simulink model "TST_VehV_DD"  (R2016b)
settings: Solver=FixedStepDiscrete  StartTime=0.0  StopTime=simTime  FixedStep=sampleTime  RelTol=1e-3
values from neighbouring files (symbols this model uses):
  testCase = 1    [initTST_VehV_DD_001.m]    (also in initTST_VehV_DD_002.m = 2)
libraries: simulink x3
settings Model: Creator=胡炎林  LastModifiedBy=胡炎林
settings DebuggingCC: SignalRangeChecking=error

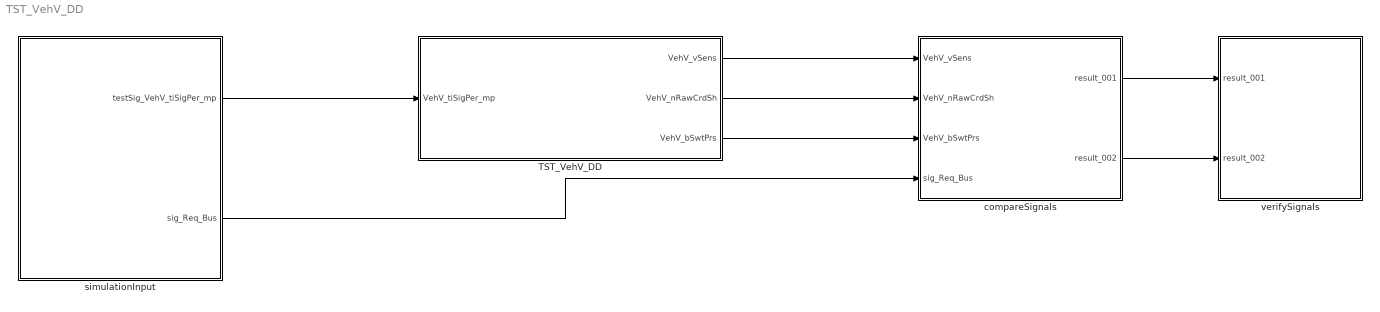
== system TST_VehV_DD ==
  TST_VehV_DD : Subsystem
  compareSignals : Subsystem
  simulationInput : Subsystem
  verifySignals : Subsystem
  wires:
  simulationInput/1(testSig_VehV_tiSigPer_mp) -> TST_VehV_DD/1(VehV_tiSigPer_mp)
  TST_VehV_DD/1(VehV_vSens) -> compareSignals/1(VehV_vSens)
  TST_VehV_DD/2(VehV_nRawCrdSh) -> compareSignals/2(VehV_nRawCrdSh)
  TST_VehV_DD/3(VehV_bSwtPrs) -> compareSignals/3(VehV_bSwtPrs)
  simulationInput/2(sig_Req_Bus) -> compareSignals/4(sig_Req_Bus)
  compareSignals/1(result_001) -> verifySignals/1(result_001)
  compareSignals/2(result_002) -> verifySignals/2(result_002)

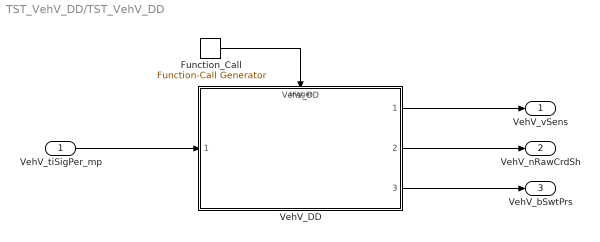
== system TST_VehV_DD/TST_VehV_DD ==
  VehV_tiSigPer_mp : Inport
  Function_Call : simulink/Ports & Subsystems/Function-Call Generator  sample_time=sampleTime  numberOfIterations=1
  VehV_DD : ModelReference  ModelNameDialog=VehV_DD  ModelReferenceVersion=1.6  TriggerPortName=function  TriggerPortTriggerType=function-call  TriggerPortStatesWhenEnabling=held
  VehV_vSens : Outport
  VehV_nRawCrdSh : Outport  Port=2
  VehV_bSwtPrs : Outport  Port=3
  wires:
  Function_Call/1 -> VehV_DD/Trigger
  VehV_tiSigPer_mp/1 -> VehV_DD/1
  VehV_DD/1 -> VehV_vSens/1
  VehV_DD/2 -> VehV_nRawCrdSh/1
  VehV_DD/3 -> VehV_bSwtPrs/1

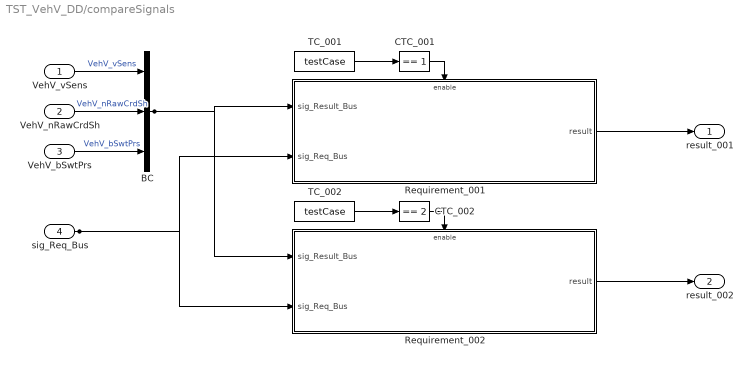
== system TST_VehV_DD/compareSignals ==
  VehV_vSens : Inport
  VehV_nRawCrdSh : Inport  Port=2
  VehV_bSwtPrs : Inport  Port=3
  sig_Req_Bus : Inport  Port=4
  BC : BusCreator  Inputs=3
  CTC_001 : simulink/Logic and Bit Operations/Compare To Constant  relop===  const=1  OutDataTypeStr=boolean
  CTC_002 : simulink/Logic and Bit Operations/Compare To Constant  relop===  const=2  OutDataTypeStr=boolean
  Requirement_001 : Subsystem
  Requirement_002 : Subsystem
  TC_001 : Constant  Value=testCase
  TC_002 : Constant  Value=testCase
  result_001 : Outport
  result_002 : Outport  Port=2
  wires:
  VehV_vSens/1 -> BC/1  "VehV_vSens"
  VehV_nRawCrdSh/1 -> BC/2  "VehV_nRawCrdSh"
  VehV_bSwtPrs/1 -> BC/3  "VehV_bSwtPrs"
  TC_001/1 -> CTC_001/1
  CTC_001/1 -> Requirement_001/Enable
  sig_Req_Bus/1 -> Requirement_001/2(sig_Req_Bus), Requirement_002/2(sig_Req_Bus)
  BC/1 -> Requirement_001/1(sig_Result_Bus), Requirement_002/1(sig_Result_Bus)
  Requirement_001/1(result) -> result_001/1
  TC_002/1 -> CTC_002/1
  CTC_002/1 -> Requirement_002/Enable
  Requirement_002/1(result) -> result_002/1

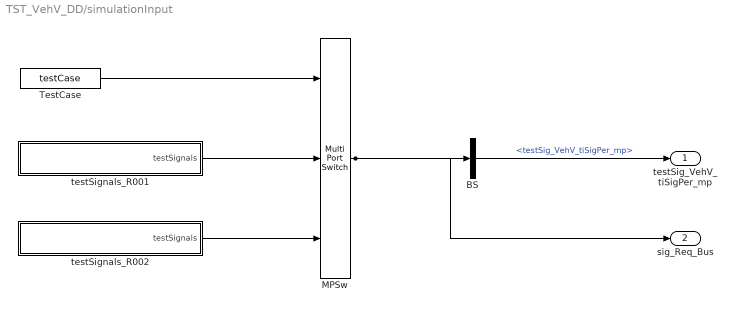
== system TST_VehV_DD/simulationInput ==
  BS : BusSelector  OutputSignals=testSig_VehV_tiSigPer_mp
  MPSw : MultiPortSwitch  Inputs=2  SaturateOnIntegerOverflow=on  InputSameDT=on
  TestCase : Constant  Value=testCase
  testSignals_R001 : Subsystem
  testSignals_R002 : Subsystem
  testSig_VehV_tiSigPer_mp : Outport
  sig_Req_Bus : Outport  Port=2
  wires:
  BS/1 -> testSig_VehV_tiSigPer_mp/1  "<testSig_VehV_tiSigPer_mp>"
  MPSw/1 -> BS/1, sig_Req_Bus/1
  TestCase/1 -> MPSw/1
  testSignals_R001/1(testSignals) -> MPSw/2
  testSignals_R002/1(testSignals) -> MPSw/3

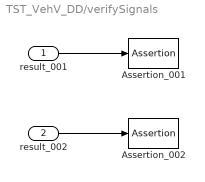
== system TST_VehV_DD/verifySignals ==
  result_001 : Inport
  result_002 : Inport  Port=2
  Assertion_001 : Assertion  Enabled=off
  Assertion_002 : Assertion  Enabled=off
  wires:
  result_001/1 -> Assertion_001/1
  result_002/1 -> Assertion_002/1

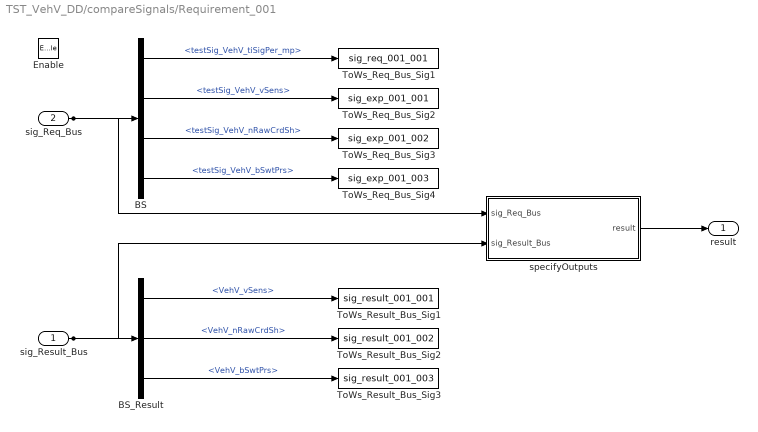
== system TST_VehV_DD/compareSignals/Requirement_001 ==
  sig_Result_Bus : Inport
  sig_Req_Bus : Inport  Port=2
  Enable : EnablePort
  BS : BusSelector  OutputSignals=testSig_VehV_tiSigPer_mp,testSig_VehV_vSens,testSig_VehV_nRawCrdSh,testSig_VehV_bSwtPrs
  BS_Result : BusSelector  OutputSignals=VehV_vSens,VehV_nRawCrdSh,VehV_bSwtPrs
  ToWs_Req_Bus_Sig1 : ToWorkspace  VariableName=sig_req_001_001  SaveFormat=Structure With Time
  ToWs_Req_Bus_Sig2 : ToWorkspace  VariableName=sig_exp_001_001  SaveFormat=Structure With Time
  ToWs_Req_Bus_Sig3 : ToWorkspace  VariableName=sig_exp_001_002  SaveFormat=Structure With Time
  ToWs_Req_Bus_Sig4 : ToWorkspace  VariableName=sig_exp_001_003  SaveFormat=Structure With Time
  ToWs_Result_Bus_Sig1 : ToWorkspace  VariableName=sig_result_001_001  SaveFormat=Structure With Time
  ToWs_Result_Bus_Sig2 : ToWorkspace  VariableName=sig_result_001_002  SaveFormat=Structure With Time
  ToWs_Result_Bus_Sig3 : ToWorkspace  VariableName=sig_result_001_003  SaveFormat=Structure With Time
  specifyOutputs : Subsystem
  result : Outport
  wires:
  sig_Req_Bus/1 -> BS/1, specifyOutputs/1(sig_Req_Bus)
  BS/1 -> ToWs_Req_Bus_Sig1/1  "<testSig_VehV_tiSigPer_mp>"
  BS/2 -> ToWs_Req_Bus_Sig2/1  "<testSig_VehV_vSens>"
  BS/3 -> ToWs_Req_Bus_Sig3/1  "<testSig_VehV_nRawCrdSh>"
  BS/4 -> ToWs_Req_Bus_Sig4/1  "<testSig_VehV_bSwtPrs>"
  sig_Result_Bus/1 -> BS_Result/1, specifyOutputs/2(sig_Result_Bus)
  BS_Result/1 -> ToWs_Result_Bus_Sig1/1  "<VehV_vSens>"
  BS_Result/2 -> ToWs_Result_Bus_Sig2/1  "<VehV_nRawCrdSh>"
  BS_Result/3 -> ToWs_Result_Bus_Sig3/1  "<VehV_bSwtPrs>"
  specifyOutputs/1(result) -> result/1

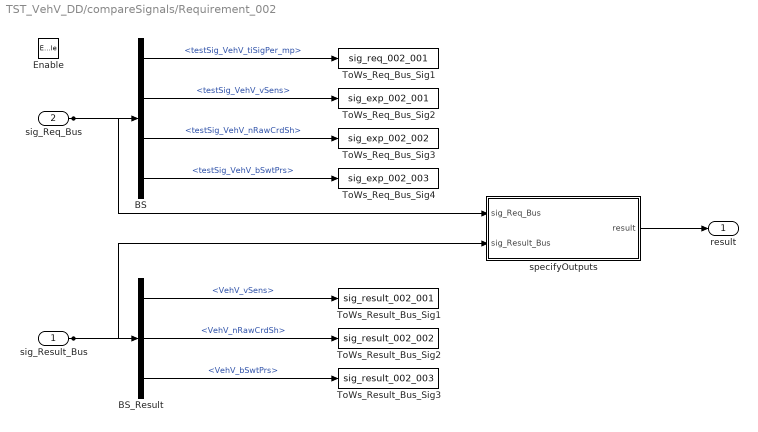
== system TST_VehV_DD/compareSignals/Requirement_002 ==
  sig_Result_Bus : Inport
  sig_Req_Bus : Inport  Port=2
  Enable : EnablePort
  BS : BusSelector  OutputSignals=testSig_VehV_tiSigPer_mp,testSig_VehV_vSens,testSig_VehV_nRawCrdSh,testSig_VehV_bSwtPrs
  BS_Result : BusSelector  OutputSignals=VehV_vSens,VehV_nRawCrdSh,VehV_bSwtPrs
  ToWs_Req_Bus_Sig1 : ToWorkspace  VariableName=sig_req_002_001  SaveFormat=Structure With Time
  ToWs_Req_Bus_Sig2 : ToWorkspace  VariableName=sig_exp_002_001  SaveFormat=Structure With Time
  ToWs_Req_Bus_Sig3 : ToWorkspace  VariableName=sig_exp_002_002  SaveFormat=Structure With Time
  ToWs_Req_Bus_Sig4 : ToWorkspace  VariableName=sig_exp_002_003  SaveFormat=Structure With Time
  ToWs_Result_Bus_Sig1 : ToWorkspace  VariableName=sig_result_002_001  SaveFormat=Structure With Time
  ToWs_Result_Bus_Sig2 : ToWorkspace  VariableName=sig_result_002_002  SaveFormat=Structure With Time
  ToWs_Result_Bus_Sig3 : ToWorkspace  VariableName=sig_result_002_003  SaveFormat=Structure With Time
  specifyOutputs : Subsystem
  result : Outport
  wires:
  sig_Req_Bus/1 -> BS/1, specifyOutputs/1(sig_Req_Bus)
  BS/1 -> ToWs_Req_Bus_Sig1/1  "<testSig_VehV_tiSigPer_mp>"
  BS/2 -> ToWs_Req_Bus_Sig2/1  "<testSig_VehV_vSens>"
  BS/3 -> ToWs_Req_Bus_Sig3/1  "<testSig_VehV_nRawCrdSh>"
  BS/4 -> ToWs_Req_Bus_Sig4/1  "<testSig_VehV_bSwtPrs>"
  sig_Result_Bus/1 -> BS_Result/1, specifyOutputs/2(sig_Result_Bus)
  BS_Result/1 -> ToWs_Result_Bus_Sig1/1  "<VehV_vSens>"
  BS_Result/2 -> ToWs_Result_Bus_Sig2/1  "<VehV_nRawCrdSh>"
  BS_Result/3 -> ToWs_Result_Bus_Sig3/1  "<VehV_bSwtPrs>"
  specifyOutputs/1(result) -> result/1

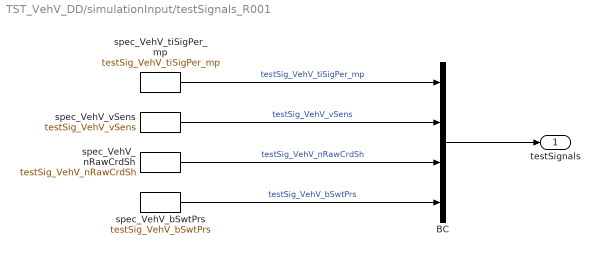
== system TST_VehV_DD/simulationInput/testSignals_R001 ==
  BC : BusCreator  Inputs=4
  spec_VehV_bSwtPrs : FromWorkspace  VariableName=testSig_VehV_bSwtPrs  Interpolate=off  OutputAfterFinalValue=Holding final value
  spec_VehV_nRawCrdSh : FromWorkspace  VariableName=testSig_VehV_nRawCrdSh  Interpolate=off  OutputAfterFinalValue=Holding final value
  spec_VehV_tiSigPer_mp : FromWorkspace  VariableName=testSig_VehV_tiSigPer_mp  Interpolate=off  OutputAfterFinalValue=Holding final value
  spec_VehV_vSens : FromWorkspace  VariableName=testSig_VehV_vSens  Interpolate=off  OutputAfterFinalValue=Holding final value
  testSignals : Outport
  wires:
  BC/1 -> testSignals/1
  spec_VehV_tiSigPer_mp/1 -> BC/1  "testSig_VehV_tiSigPer_mp"
  spec_VehV_vSens/1 -> BC/2  "testSig_VehV_vSens"
  spec_VehV_nRawCrdSh/1 -> BC/3  "testSig_VehV_nRawCrdSh"
  spec_VehV_bSwtPrs/1 -> BC/4  "testSig_VehV_bSwtPrs"

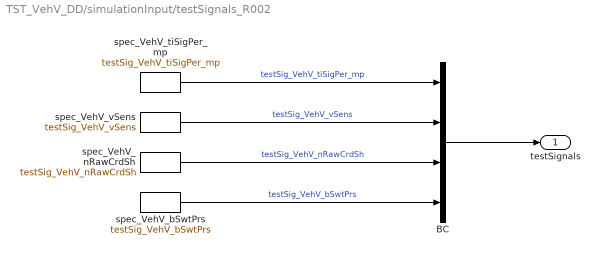
== system TST_VehV_DD/simulationInput/testSignals_R002 ==
  BC : BusCreator  Inputs=4
  spec_VehV_bSwtPrs : FromWorkspace  VariableName=testSig_VehV_bSwtPrs  Interpolate=off  OutputAfterFinalValue=Holding final value
  spec_VehV_nRawCrdSh : FromWorkspace  VariableName=testSig_VehV_nRawCrdSh  Interpolate=off  OutputAfterFinalValue=Holding final value
  spec_VehV_tiSigPer_mp : FromWorkspace  VariableName=testSig_VehV_tiSigPer_mp  Interpolate=off  OutputAfterFinalValue=Holding final value
  spec_VehV_vSens : FromWorkspace  VariableName=testSig_VehV_vSens  Interpolate=off  OutputAfterFinalValue=Holding final value
  testSignals : Outport
  wires:
  BC/1 -> testSignals/1
  spec_VehV_tiSigPer_mp/1 -> BC/1  "testSig_VehV_tiSigPer_mp"
  spec_VehV_vSens/1 -> BC/2  "testSig_VehV_vSens"
  spec_VehV_nRawCrdSh/1 -> BC/3  "testSig_VehV_nRawCrdSh"
  spec_VehV_bSwtPrs/1 -> BC/4  "testSig_VehV_bSwtPrs"

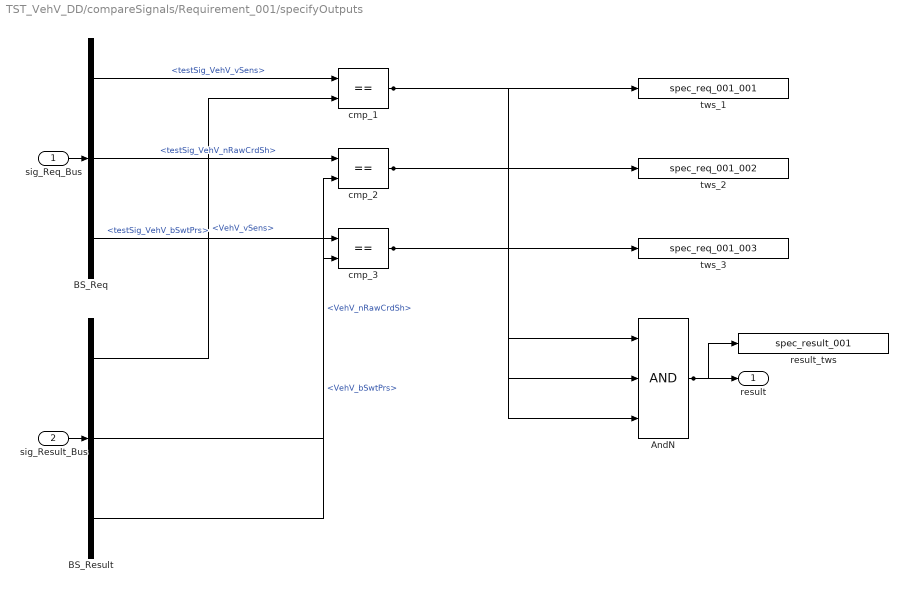
== system TST_VehV_DD/compareSignals/Requirement_001/specifyOutputs ==
  sig_Req_Bus : Inport
  sig_Result_Bus : Inport  Port=2
  AndN : Logic  Inputs=3
  BS_Req : BusSelector  OutputSignals=testSig_VehV_vSens,testSig_VehV_nRawCrdSh,testSig_VehV_bSwtPrs
  BS_Result : BusSelector  OutputSignals=VehV_vSens,VehV_nRawCrdSh,VehV_bSwtPrs
  cmp_1 : RelationalOperator  Operator===  RndMeth=Nearest  InputSameDT=on
  cmp_2 : RelationalOperator  Operator===  RndMeth=Nearest  InputSameDT=on
  cmp_3 : RelationalOperator  Operator===  RndMeth=Nearest  InputSameDT=on
  result_tws : ToWorkspace  VariableName=spec_result_001
  tws_1 : ToWorkspace  VariableName=spec_req_001_001
  tws_2 : ToWorkspace  VariableName=spec_req_001_002
  tws_3 : ToWorkspace  VariableName=spec_req_001_003
  result : Outport
  wires:
  sig_Req_Bus/1 -> BS_Req/1
  sig_Result_Bus/1 -> BS_Result/1
  AndN/1 -> result/1, result_tws/1
  BS_Req/1 -> cmp_1/1  "<testSig_VehV_vSens>"
  BS_Result/1 -> cmp_1/2  "<VehV_vSens>"
  cmp_1/1 -> tws_1/1, AndN/1
  BS_Req/2 -> cmp_2/1  "<testSig_VehV_nRawCrdSh>"
  BS_Result/2 -> cmp_2/2  "<VehV_nRawCrdSh>"
  cmp_2/1 -> tws_2/1, AndN/2
  BS_Req/3 -> cmp_3/1  "<testSig_VehV_bSwtPrs>"
  BS_Result/3 -> cmp_3/2  "<VehV_bSwtPrs>"
  cmp_3/1 -> tws_3/1, AndN/3

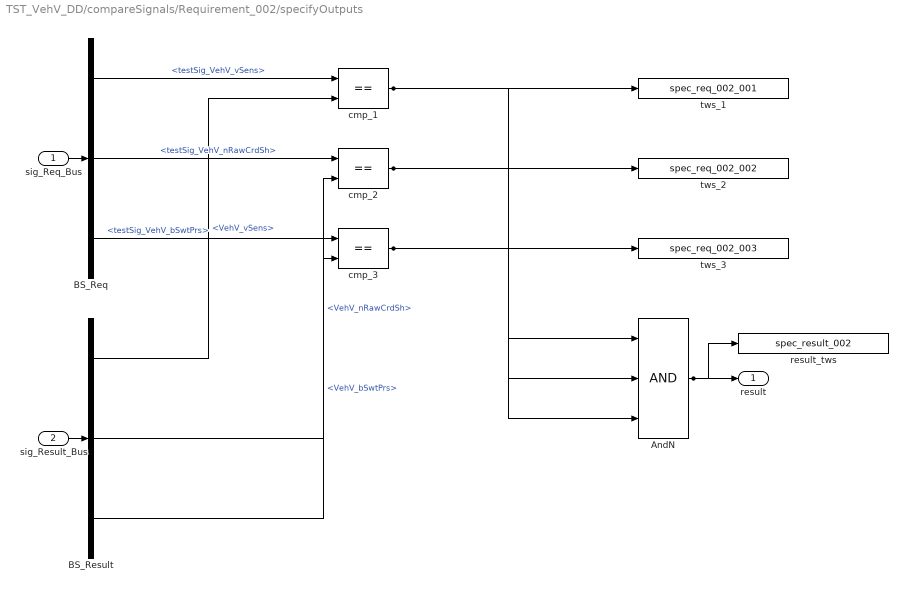
== system TST_VehV_DD/compareSignals/Requirement_002/specifyOutputs ==
  sig_Req_Bus : Inport
  sig_Result_Bus : Inport  Port=2
  AndN : Logic  Inputs=3
  BS_Req : BusSelector  OutputSignals=testSig_VehV_vSens,testSig_VehV_nRawCrdSh,testSig_VehV_bSwtPrs
  BS_Result : BusSelector  OutputSignals=VehV_vSens,VehV_nRawCrdSh,VehV_bSwtPrs
  cmp_1 : RelationalOperator  Operator===  RndMeth=Nearest  InputSameDT=on
  cmp_2 : RelationalOperator  Operator===  RndMeth=Nearest  InputSameDT=on
  cmp_3 : RelationalOperator  Operator===  RndMeth=Nearest  InputSameDT=on
  result_tws : ToWorkspace  VariableName=spec_result_002
  tws_1 : ToWorkspace  VariableName=spec_req_002_001
  tws_2 : ToWorkspace  VariableName=spec_req_002_002
  tws_3 : ToWorkspace  VariableName=spec_req_002_003
  result : Outport
  wires:
  sig_Req_Bus/1 -> BS_Req/1
  sig_Result_Bus/1 -> BS_Result/1
  AndN/1 -> result/1, result_tws/1
  BS_Req/1 -> cmp_1/1  "<testSig_VehV_vSens>"
  BS_Result/1 -> cmp_1/2  "<VehV_vSens>"
  cmp_1/1 -> tws_1/1, AndN/1
  BS_Req/2 -> cmp_2/1  "<testSig_VehV_nRawCrdSh>"
  BS_Result/2 -> cmp_2/2  "<VehV_nRawCrdSh>"
  cmp_2/1 -> tws_2/1, AndN/2
  BS_Req/3 -> cmp_3/1  "<testSig_VehV_bSwtPrs>"
  BS_Result/3 -> cmp_3/2  "<VehV_bSwtPrs>"
  cmp_3/1 -> tws_3/1, AndN/3
